simulink model "esercizio4S"  (R2020a)
settings: Solver=VariableStepAuto  StartTime=0.0  StopTime=50.0  RelTol=1e-3
values from neighbouring files (symbols this model uses):
  K = place(A, B, P)    [esempio0.m]    (also in esercizio.m; esercizio2.m; esercizio3.m; esercizio4.m)
settings Model: Creator=itama  LastModifiedBy=itama

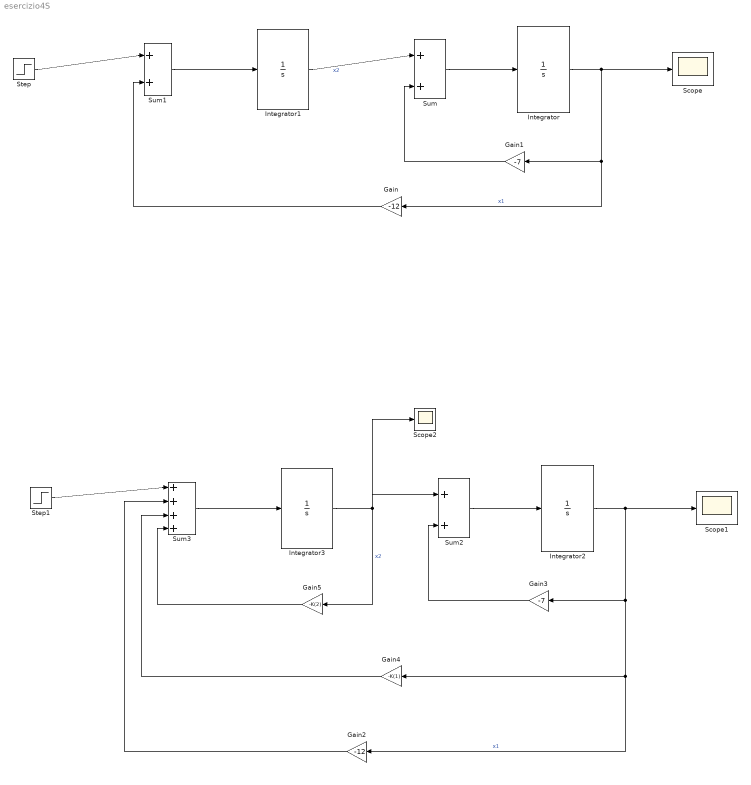
== system esercizio4S ==
  Gain : Gain  Gain=-12
  Gain1 : Gain  Gain=-7
  Gain2 : Gain  Gain=-12
  Gain3 : Gain  Gain=-7
  Gain4 : Gain  Gain=-K(1)
  Gain5 : Gain  Gain=-K(2)
  Integrator{,1..3} (4 alike) : Integrator
  Scope : Scope
  Scope1 : Scope
  Scope2 : Scope
  Step : Step  SampleTime=0
  Step1 : Step  SampleTime=0
  Sum : Sum  Inputs=|++
  Sum1 : Sum  Inputs=|++
  Sum2 : Sum  Inputs=|++
  Sum3 : Sum  Inputs=|++++
  wires:
  Integrator/1 -> Gain/1, Gain1/1, Scope/1  "x1"
  Sum/1 -> Integrator/1
  Gain1/1 -> Sum/2
  Integrator1/1 -> Sum/1  "x2"
  Sum1/1 -> Integrator1/1
  Gain/1 -> Sum1/2
  Step/1 -> Sum1/1
  Gain2/1 -> Sum3/2
  Gain3/1 -> Sum2/2
  Integrator2/1 -> Gain2/1, Gain4/1, Gain3/1, Scope1/1  "x1"
  Sum2/1 -> Integrator2/1
  Integrator3/1 -> Scope2/1, Sum2/1, Gain5/1  "x2"
  Step1/1 -> Sum3/1
  Sum3/1 -> Integrator3/1
  Gain4/1 -> Sum3/3
  Gain5/1 -> Sum3/4
